simulink model "decoder_debug"  (R2020b)
settings: Solver=VariableStepAuto  StartTime=0.0  StopTime=10.0  RelTol=1e-3
libraries: eeQuadratureDecoder x1
settings Model: Creator=kjartan  LastModifiedBy=kjartan

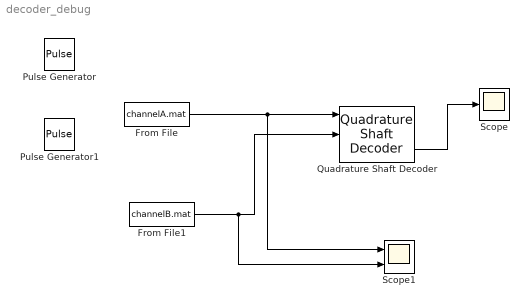
== system decoder_debug ==
  From File : FromFile  FileName=channelA.mat  SampleTime=0
  From File1 : FromFile  FileName=channelB.mat  SampleTime=0
  Pulse Generator : DiscretePulseGenerator  PulseType=Time based  Amplitude=5  Period=1  PulseWidth=50
  Pulse Generator1 : DiscretePulseGenerator  PulseType=Time based  Amplitude=5  Period=1  PulseWidth=50  PhaseDelay=0.25
  Quadrature Shaft Decoder : eeQuadratureDecoder/Quadrature Shaft Decoder  NPulse=4  Ts=1e-2
      settings: SourceProductBaseCode=PS
  Scope : Scope
  Scope1 : Scope  NumInputPorts=2
  wires:
  From File1/1 -> Scope1/2, Quadrature Shaft Decoder/2
  From File/1 -> Scope1/1, Quadrature Shaft Decoder/1
  Quadrature Shaft Decoder/2 -> Scope/1
